simulink model "attsync2"  (R2013a)
settings: Solver=ode45  StartTime=0.0  StopTime=30  RelTol=1e-3
settings Model: Creator=daqing_yi  LastModifiedBy=daqing_yi
settings DataIOCC: SignalLoggingSaveFormat=ModelDataLogs
settings DebuggingCC: MultiTaskDSMMsg=warning  MultiTaskCondExecSysMsg=none  StrictBusMsg=None
settings RTWCC: IncludeERTFirstTime=on

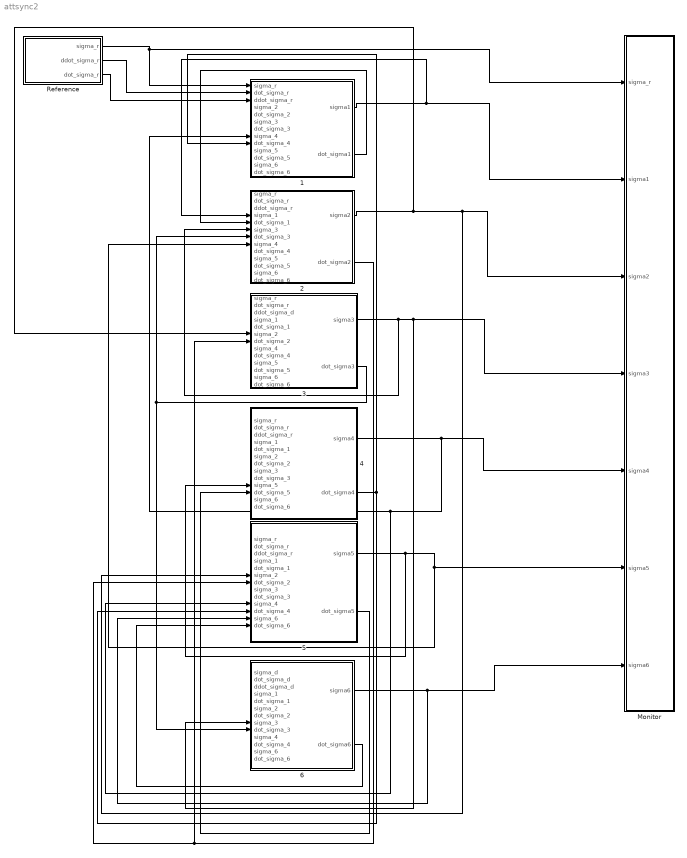
== system attsync2 ==
  1 : Subsystem
  2 : Subsystem
  3 : Subsystem
  4 : Subsystem
  5 : Subsystem
  6 : Subsystem
  Monitor : Subsystem
  Reference : Subsystem
  wires:
  Reference/1(sigma_r) -> 1/1(sigma_r), Monitor/1(sigma_r)
  1/1(sigma1) -> 2/4(sigma_1), Monitor/2(sigma1)
  2/1(sigma2) -> 3/6(sigma_2), 5/6(sigma_2), Monitor/3(sigma2)
  3/1(sigma3) -> 6/8(sigma_3), Monitor/4(sigma3), 2/6(sigma_3)
  4/1(sigma4) -> Monitor/5(sigma4), 5/10(sigma_4), 1/8(sigma_4)
  5/1(sigma5) -> 2/8(sigma_4), Monitor/6(sigma5), 4/10(sigma_5)
  Reference/2(ddot_sigma_r) -> 1/2(dot_sigma_r)
  Reference/3(dot_sigma_r) -> 1/3(ddot_sigma_r)
  6/1(sigma6) -> Monitor/7(sigma6), 5/12(sigma_6)
  6/2(dot_sigma6) -> 5/13(dot_sigma_6)
  3/2(dot_sigma3) -> 6/9(dot_sigma_3), 2/7(dot_sigma_3)
  4/2(dot_sigma4) -> 1/9(dot_sigma_4), 5/11(dot_sigma_4)
  5/2(dot_sigma5) -> 4/11(dot_sigma_5)
  2/2(dot_sigma2) -> 3/7(dot_sigma_2), 5/7(dot_sigma_2)
  1/2(dot_sigma1) -> 2/5(dot_sigma_1)

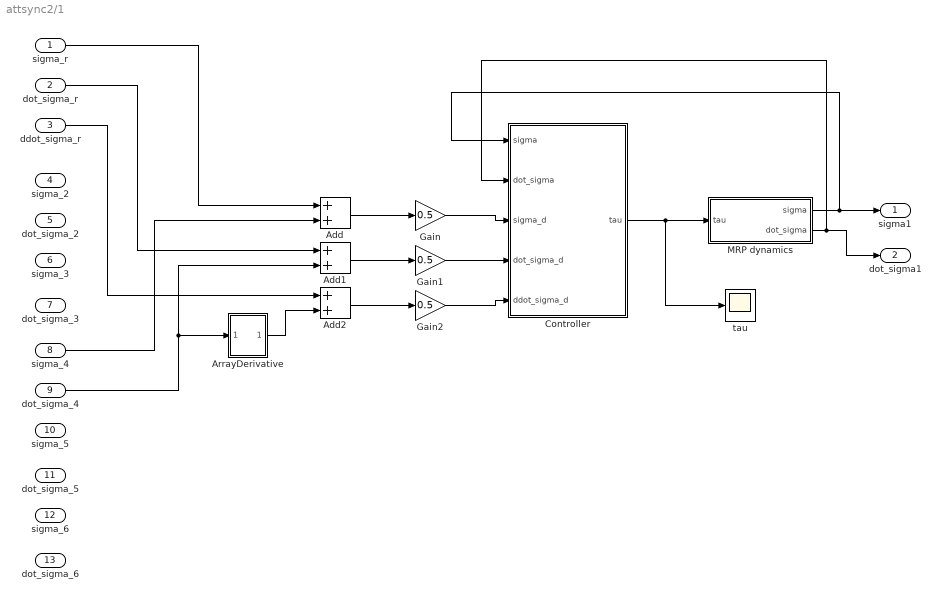
== system attsync2/1 ==
  sigma_r : Inport
  dot_sigma_r : Inport  Port=2
  ddot_sigma_r : Inport  Port=3
  sigma_2 : Inport  Port=4  PortDimensions=3
  dot_sigma_2 : Inport  Port=5  PortDimensions=3
  sigma_3 : Inport  Port=6  PortDimensions=3
  dot_sigma_3 : Inport  Port=7  PortDimensions=3
  sigma_4 : Inport  Port=8  PortDimensions=3
  dot_sigma_4 : Inport  Port=9  PortDimensions=3
  sigma_5 : Inport  Port=10  PortDimensions=3
  dot_sigma_5 : Inport  Port=11  PortDimensions=3
  sigma_6 : Inport  Port=12  PortDimensions=3
  dot_sigma_6 : Inport  Port=13  PortDimensions=3
  Add : Sum
  Add1 : Sum
  Add2 : Sum
  ArrayDerivative : Subsystem
  Controller : Subsystem
  Gain : Gain  Gain=0.5
  Gain1 : Gain  Gain=0.5
  Gain2 : Gain  Gain=0.5
  MRP dynamics : Subsystem
  tau : Scope
  sigma1 : Outport
  dot_sigma1 : Outport  Port=2
  wires:
  Controller/1(tau) -> tau/1, MRP dynamics/1(tau)
  MRP dynamics/1(sigma) -> sigma1/1, Controller/1(sigma)
  MRP dynamics/2(dot_sigma) -> dot_sigma1/1, Controller/2(dot_sigma)
  Add/1 -> Gain/1
  Add1/1 -> Gain1/1
  Add2/1 -> Gain2/1
  Gain/1 -> Controller/3(sigma_d)
  Gain1/1 -> Controller/4(dot_sigma_d)
  Gain2/1 -> Controller/5(ddot_sigma_d)
  sigma_r/1 -> Add/1
  dot_sigma_r/1 -> Add1/1
  ddot_sigma_r/1 -> Add2/1
  sigma_4/1 -> Add/2
  dot_sigma_4/1 -> Add1/2, ArrayDerivative/1(In1)
  ArrayDerivative/1(Out1) -> Add2/2

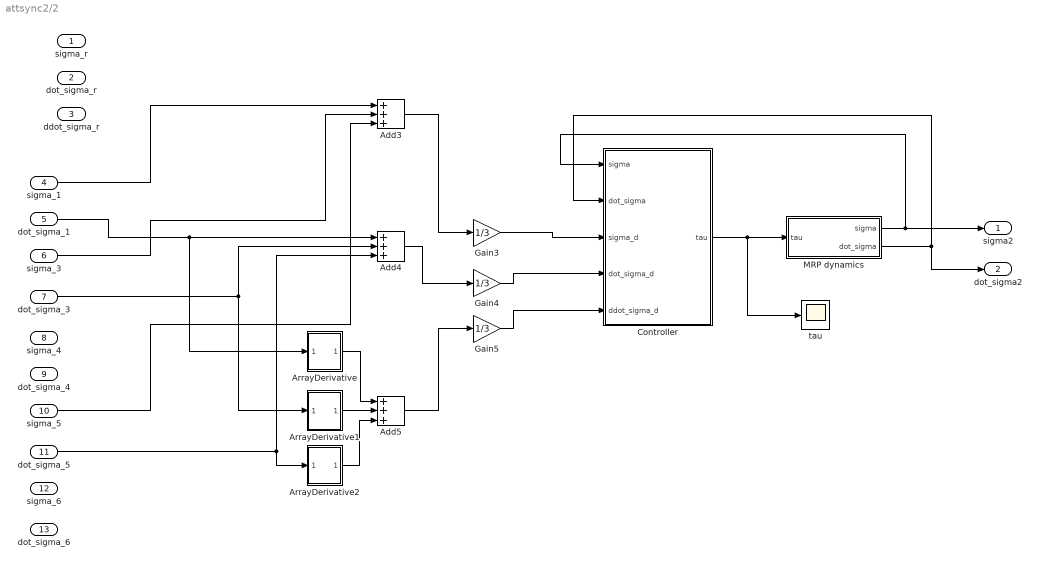
== system attsync2/2 ==
  sigma_r : Inport
  dot_sigma_r : Inport  Port=2
  ddot_sigma_r : Inport  Port=3
  sigma_1 : Inport  Port=4  PortDimensions=3
  dot_sigma_1 : Inport  Port=5  PortDimensions=3
  sigma_3 : Inport  Port=6  PortDimensions=3
  dot_sigma_3 : Inport  Port=7  PortDimensions=3
  sigma_4 : Inport  Port=8  PortDimensions=3
  dot_sigma_4 : Inport  Port=9  PortDimensions=3
  sigma_5 : Inport  Port=10  PortDimensions=3
  dot_sigma_5 : Inport  Port=11  PortDimensions=3
  sigma_6 : Inport  Port=12  PortDimensions=3
  dot_sigma_6 : Inport  Port=13  PortDimensions=3
  Add3 : Sum  Inputs=+++
  Add4 : Sum  Inputs=+++
  Add5 : Sum  Inputs=+++
  ArrayDerivative : Subsystem
  ArrayDerivative1 : Subsystem
  ArrayDerivative2 : Subsystem
  Controller : Subsystem
  Gain3 : Gain  Gain=1/3
  Gain4 : Gain  Gain=1/3
  Gain5 : Gain  Gain=1/3
  MRP dynamics : Subsystem
  tau : Scope
  sigma2 : Outport
  dot_sigma2 : Outport  Port=2
  wires:
  Controller/1(tau) -> tau/1, MRP dynamics/1(tau)
  MRP dynamics/1(sigma) -> sigma2/1, Controller/1(sigma)
  MRP dynamics/2(dot_sigma) -> dot_sigma2/1, Controller/2(dot_sigma)
  Add4/1 -> Gain4/1
  Add3/1 -> Gain3/1
  Gain3/1 -> Controller/3(sigma_d)
  Gain4/1 -> Controller/4(dot_sigma_d)
  Add5/1 -> Gain5/1
  Gain5/1 -> Controller/5(ddot_sigma_d)
  sigma_1/1 -> Add3/1
  sigma_3/1 -> Add3/2
  sigma_5/1 -> Add3/3
  dot_sigma_5/1 -> ArrayDerivative2/1(In1), Add4/3
  dot_sigma_1/1 -> ArrayDerivative/1(In1), Add4/1
  dot_sigma_3/1 -> ArrayDerivative1/1(In1), Add4/2
  ArrayDerivative2/1(Out1) -> Add5/3
  ArrayDerivative1/1(Out1) -> Add5/2
  ArrayDerivative/1(Out1) -> Add5/1

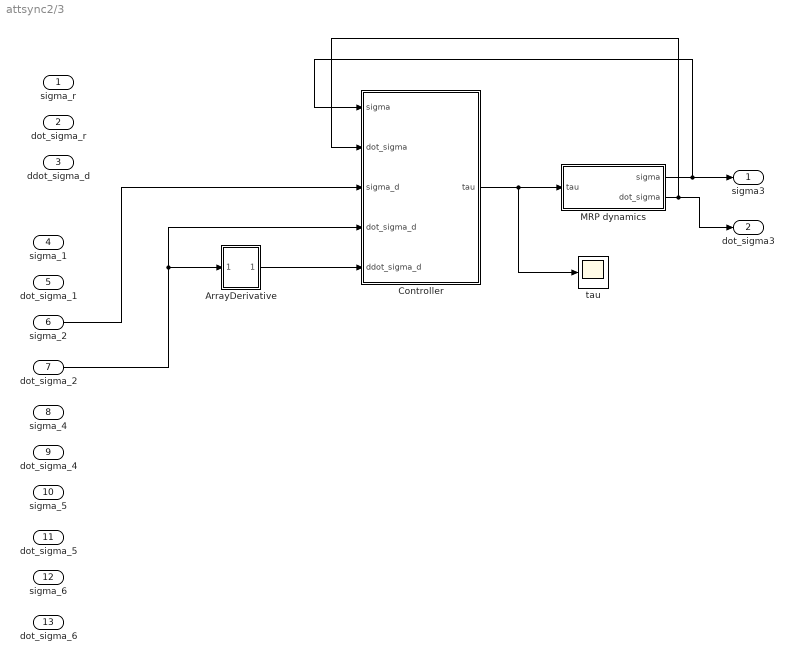
== system attsync2/3 ==
  sigma_r : Inport
  dot_sigma_r : Inport  Port=2
  ddot_sigma_d : Inport  Port=3
  sigma_1 : Inport  Port=4  PortDimensions=3
  dot_sigma_1 : Inport  Port=5  PortDimensions=3
  sigma_2 : Inport  Port=6  PortDimensions=3
  dot_sigma_2 : Inport  Port=7  PortDimensions=3
  sigma_4 : Inport  Port=8  PortDimensions=3
  dot_sigma_4 : Inport  Port=9  PortDimensions=3
  sigma_5 : Inport  Port=10  PortDimensions=3
  dot_sigma_5 : Inport  Port=11  PortDimensions=3
  sigma_6 : Inport  Port=12  PortDimensions=3
  dot_sigma_6 : Inport  Port=13  PortDimensions=3
  ArrayDerivative : Subsystem
  Controller : Subsystem
  MRP dynamics : Subsystem
  tau : Scope
  sigma3 : Outport
  dot_sigma3 : Outport  Port=2
  wires:
  Controller/1(tau) -> tau/1, MRP dynamics/1(tau)
  MRP dynamics/1(sigma) -> sigma3/1, Controller/1(sigma)
  MRP dynamics/2(dot_sigma) -> dot_sigma3/1, Controller/2(dot_sigma)
  sigma_2/1 -> Controller/3(sigma_d)
  dot_sigma_2/1 -> ArrayDerivative/1(In1), Controller/4(dot_sigma_d)
  ArrayDerivative/1(Out1) -> Controller/5(ddot_sigma_d)

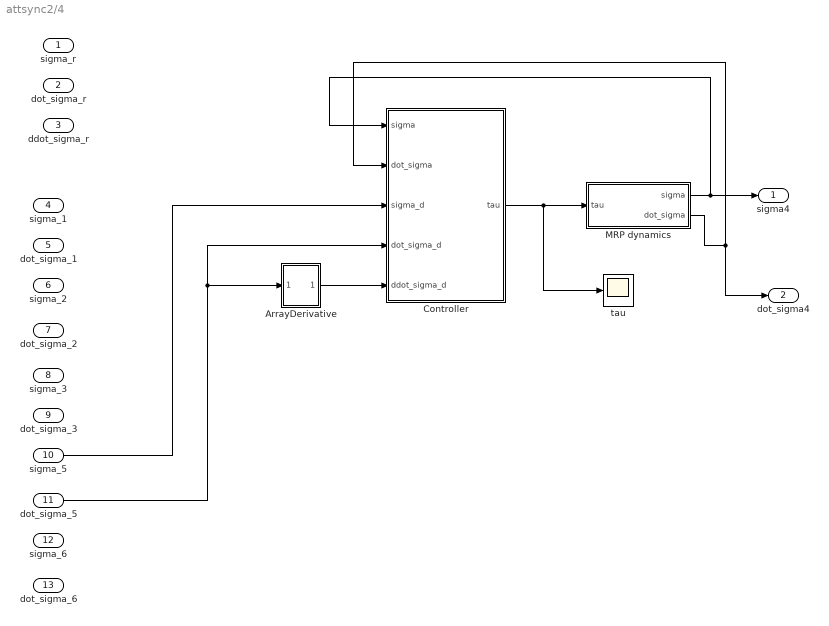
== system attsync2/4 ==
  sigma_r : Inport
  dot_sigma_r : Inport  Port=2
  ddot_sigma_r : Inport  Port=3
  sigma_1 : Inport  Port=4  PortDimensions=3
  dot_sigma_1 : Inport  Port=5  PortDimensions=3
  sigma_2 : Inport  Port=6  PortDimensions=3
  dot_sigma_2 : Inport  Port=7  PortDimensions=3
  sigma_3 : Inport  Port=8  PortDimensions=3
  dot_sigma_3 : Inport  Port=9  PortDimensions=3
  sigma_5 : Inport  Port=10  PortDimensions=3
  dot_sigma_5 : Inport  Port=11  PortDimensions=3
  sigma_6 : Inport  Port=12  PortDimensions=3
  dot_sigma_6 : Inport  Port=13  PortDimensions=3
  ArrayDerivative : Subsystem
  Controller : Subsystem
  MRP dynamics : Subsystem
  tau : Scope
  sigma4 : Outport
  dot_sigma4 : Outport  Port=2
  wires:
  Controller/1(tau) -> tau/1, MRP dynamics/1(tau)
  MRP dynamics/1(sigma) -> sigma4/1, Controller/1(sigma)
  MRP dynamics/2(dot_sigma) -> Controller/2(dot_sigma), dot_sigma4/1
  sigma_5/1 -> Controller/3(sigma_d)
  dot_sigma_5/1 -> ArrayDerivative/1(In1), Controller/4(dot_sigma_d)
  ArrayDerivative/1(Out1) -> Controller/5(ddot_sigma_d)

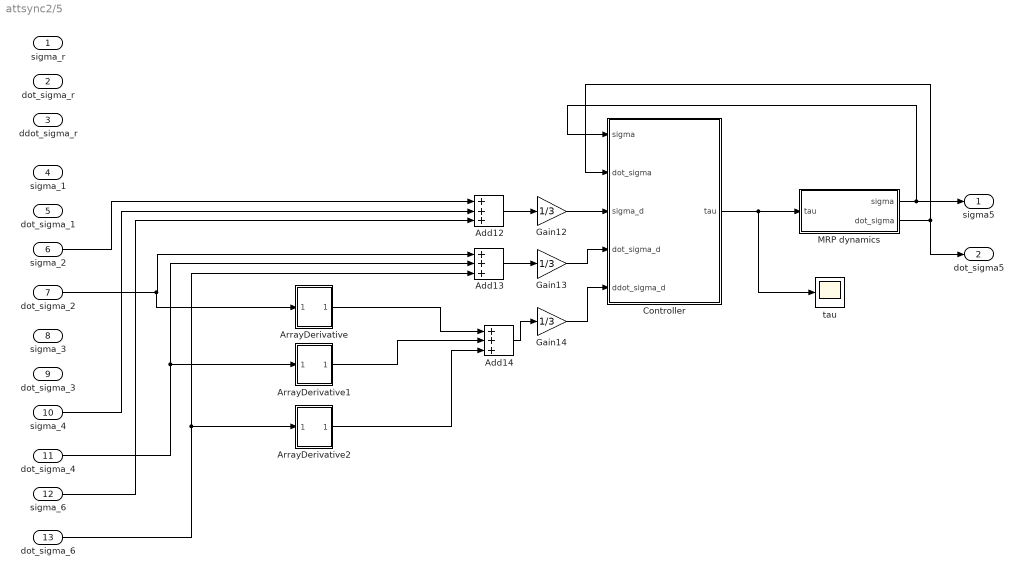
== system attsync2/5 ==
  sigma_r : Inport
  dot_sigma_r : Inport  Port=2
  ddot_sigma_r : Inport  Port=3
  sigma_1 : Inport  Port=4  PortDimensions=3
  dot_sigma_1 : Inport  Port=5  PortDimensions=3
  sigma_2 : Inport  Port=6  PortDimensions=3
  dot_sigma_2 : Inport  Port=7  PortDimensions=3
  sigma_3 : Inport  Port=8  PortDimensions=3
  dot_sigma_3 : Inport  Port=9  PortDimensions=3
  sigma_4 : Inport  Port=10  PortDimensions=3
  dot_sigma_4 : Inport  Port=11  PortDimensions=3
  sigma_6 : Inport  Port=12  PortDimensions=3
  dot_sigma_6 : Inport  Port=13  PortDimensions=3
  Add12 : Sum  Inputs=+++
  Add13 : Sum  Inputs=+++
  Add14 : Sum  Inputs=+++
  ArrayDerivative : Subsystem
  ArrayDerivative1 : Subsystem
  ArrayDerivative2 : Subsystem
  Controller : Subsystem
  Gain12 : Gain  Gain=1/3
  Gain13 : Gain  Gain=1/3
  Gain14 : Gain  Gain=1/3
  MRP dynamics : Subsystem
  tau : Scope
  sigma5 : Outport
  dot_sigma5 : Outport  Port=2
  wires:
  Controller/1(tau) -> tau/1, MRP dynamics/1(tau)
  MRP dynamics/1(sigma) -> sigma5/1, Controller/1(sigma)
  MRP dynamics/2(dot_sigma) -> dot_sigma5/1, Controller/2(dot_sigma)
  Add12/1 -> Gain12/1
  Add13/1 -> Gain13/1
  Add14/1 -> Gain14/1
  Gain12/1 -> Controller/3(sigma_d)
  Gain13/1 -> Controller/4(dot_sigma_d)
  Gain14/1 -> Controller/5(ddot_sigma_d)
  sigma_2/1 -> Add12/1
  sigma_4/1 -> Add12/2
  sigma_6/1 -> Add12/3
  dot_sigma_2/1 -> ArrayDerivative/1(In1), Add13/1
  dot_sigma_4/1 -> ArrayDerivative1/1(In1), Add13/2
  dot_sigma_6/1 -> ArrayDerivative2/1(In1), Add13/3
  ArrayDerivative1/1(Out1) -> Add14/2
  ArrayDerivative2/1(Out1) -> Add14/3
  ArrayDerivative/1(Out1) -> Add14/1

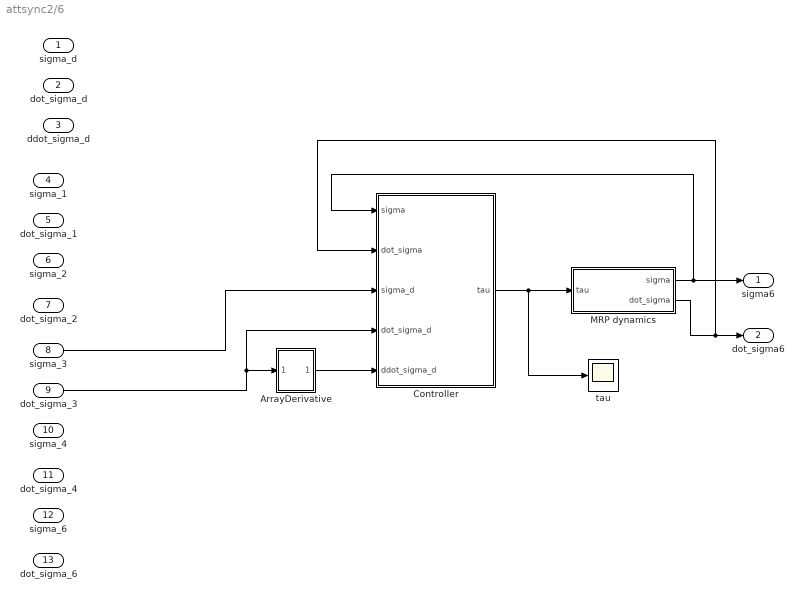
== system attsync2/6 ==
  sigma_d : Inport
  dot_sigma_d : Inport  Port=2
  ddot_sigma_d : Inport  Port=3
  sigma_1 : Inport  Port=4  PortDimensions=3
  dot_sigma_1 : Inport  Port=5  PortDimensions=3
  sigma_2 : Inport  Port=6  PortDimensions=3
  dot_sigma_2 : Inport  Port=7  PortDimensions=3
  sigma_3 : Inport  Port=8  PortDimensions=3
  dot_sigma_3 : Inport  Port=9  PortDimensions=3
  sigma_4 : Inport  Port=10  PortDimensions=3
  dot_sigma_4 : Inport  Port=11  PortDimensions=3
  sigma_6 : Inport  Port=12  PortDimensions=3
  dot_sigma_6 : Inport  Port=13  PortDimensions=3
  ArrayDerivative : Subsystem
  Controller : Subsystem
  MRP dynamics : Subsystem
  tau : Scope
  sigma6 : Outport
  dot_sigma6 : Outport  Port=2
  wires:
  Controller/1(tau) -> tau/1, MRP dynamics/1(tau)
  MRP dynamics/1(sigma) -> sigma6/1, Controller/1(sigma)
  MRP dynamics/2(dot_sigma) -> Controller/2(dot_sigma), dot_sigma6/1
  sigma_3/1 -> Controller/3(sigma_d)
  dot_sigma_3/1 -> ArrayDerivative/1(In1), Controller/4(dot_sigma_d)
  ArrayDerivative/1(Out1) -> Controller/5(ddot_sigma_d)

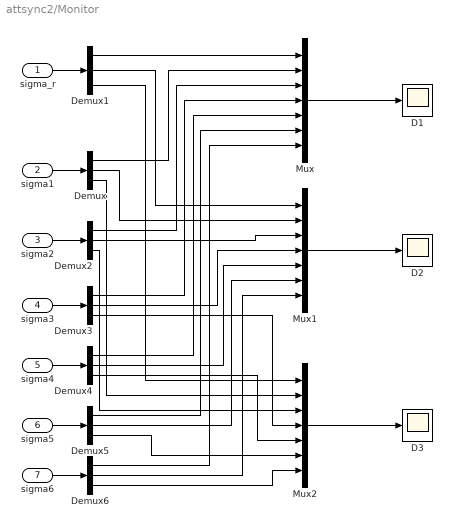
== system attsync2/Monitor ==
  sigma_r : Inport
  sigma1 : Inport  Port=2
  sigma2 : Inport  Port=3
  sigma3 : Inport  Port=4
  sigma4 : Inport  Port=5
  sigma5 : Inport  Port=6
  sigma6 : Inport  Port=7
  D1 : Scope
      settings: YMin=-8  YMax=1.5  SaveName=D1
  D2 : Scope
      settings: SaveName=D2
  D3 : Scope
      settings: SaveName=D3
  Demux{,1..6} (7 alike) : Demux  Outputs=3
  Mux : Mux  Inputs=7
  Mux1 : Mux  Inputs=7
  Mux2 : Mux  Inputs=7
  wires:
  sigma1/1 -> Demux/1
  sigma_r/1 -> Demux1/1
  Demux1/1 -> Mux/1
  Mux/1 -> D1/1
  Mux1/1 -> D2/1
  Mux2/1 -> D3/1
  sigma3/1 -> Demux3/1
  sigma4/1 -> Demux4/1
  sigma5/1 -> Demux5/1
  sigma6/1 -> Demux6/1
  sigma2/1 -> Demux2/1
  Demux1/2 -> Mux1/1
  Demux1/3 -> Mux2/1
  Demux/1 -> Mux/2
  Demux2/1 -> Mux/3
  Demux3/1 -> Mux/4
  Demux4/1 -> Mux/5
  Demux5/1 -> Mux/6
  Demux6/1 -> Mux/7
  Demux/2 -> Mux1/2
  Demux2/2 -> Mux1/3
  Demux3/2 -> Mux1/4
  Demux4/2 -> Mux1/5
  Demux5/2 -> Mux1/6
  Demux6/2 -> Mux1/7
  Demux/3 -> Mux2/2
  Demux2/3 -> Mux2/3
  Demux3/3 -> Mux2/4
  Demux4/3 -> Mux2/5
  Demux5/3 -> Mux2/6
  Demux6/3 -> Mux2/7

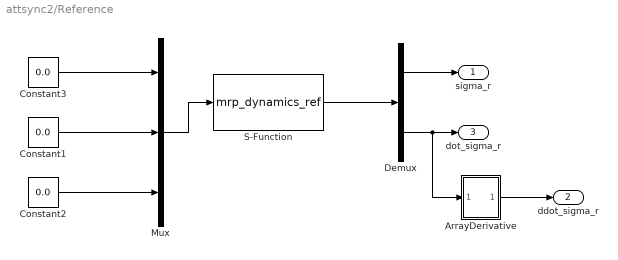
== system attsync2/Reference ==
  ArrayDerivative : Subsystem
  Constant1 : Constant  Value=0.0
  Constant2 : Constant  Value=0.0
  Constant3 : Constant  Value=0.0
  Demux : Demux  Outputs=2
  Mux : Mux  Inputs=3
  S-Function : S-Function  FunctionName=mrp_dynamics_ref  EnableBusSupport=off
  sigma_r : Outport  PortDimensions=3
  ddot_sigma_r : Outport  Port=2
  dot_sigma_r : Outport  Port=3
  wires:
  Constant3/1 -> Mux/1
  Constant1/1 -> Mux/2
  Constant2/1 -> Mux/3
  Mux/1 -> S-Function/1
  S-Function/1 -> Demux/1
  Demux/1 -> sigma_r/1
  Demux/2 -> ArrayDerivative/1(In1), dot_sigma_r/1
  ArrayDerivative/1(Out1) -> ddot_sigma_r/1

== system attsync2/1/ArrayDerivative ==
  In1 : Inport
  Demux : Demux  Outputs=3
  Derivative : Derivative
  Derivative1 : Derivative
  Derivative2 : Derivative
  Mux : Mux  Inputs=3
  Out1 : Outport
  wires:
  Mux/1 -> Out1/1
  In1/1 -> Demux/1
  Derivative1/1 -> Mux/2
  Demux/2 -> Derivative1/1
  Derivative2/1 -> Mux/3
  Demux/3 -> Derivative2/1
  Demux/1 -> Derivative/1
  Derivative/1 -> Mux/1

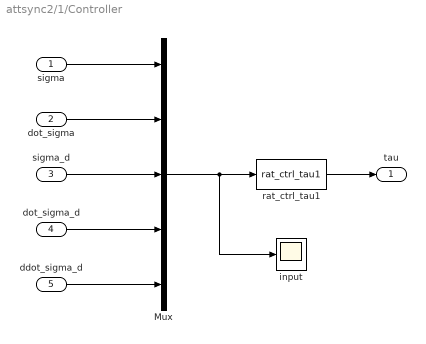
== system attsync2/1/Controller ==
  sigma : Inport
  dot_sigma : Inport  Port=2
  sigma_d : Inport  Port=3
  dot_sigma_d : Inport  Port=4
  ddot_sigma_d : Inport  Port=5
  Mux : Mux  Inputs=5
  input : Scope
      settings: SaveName=ScopeData4
  rat_ctrl_tau1 : MATLABFcn  MATLABFcn=rat_ctrl_tau1  OutputDimensions=3
  tau : Outport
  wires:
  sigma/1 -> Mux/1
  sigma_d/1 -> Mux/3
  Mux/1 -> input/1, rat_ctrl_tau1/1
  dot_sigma/1 -> Mux/2
  rat_ctrl_tau1/1 -> tau/1
  dot_sigma_d/1 -> Mux/4
  ddot_sigma_d/1 -> Mux/5

== system attsync2/1/MRP dynamics ==
  tau : Inport
  Demux : Demux  Outputs=2
  S-Function : S-Function  FunctionName=mrp_dynamics1  EnableBusSupport=off
  sigma : Outport  PortDimensions=3
  dot_sigma : Outport  Port=2  PortDimensions=3
  wires:
  tau/1 -> S-Function/1
  Demux/1 -> sigma/1
  Demux/2 -> dot_sigma/1
  S-Function/1 -> Demux/1

== system attsync2/2/ArrayDerivative ==
  In1 : Inport
  Demux : Demux  Outputs=3
  Derivative : Derivative
  Derivative1 : Derivative
  Derivative2 : Derivative
  Mux : Mux  Inputs=3
  Out1 : Outport
  wires:
  Mux/1 -> Out1/1
  In1/1 -> Demux/1
  Derivative1/1 -> Mux/2
  Demux/2 -> Derivative1/1
  Derivative2/1 -> Mux/3
  Demux/3 -> Derivative2/1
  Demux/1 -> Derivative/1
  Derivative/1 -> Mux/1

== system attsync2/2/ArrayDerivative1 ==
  In1 : Inport
  Demux : Demux  Outputs=3
  Derivative : Derivative
  Derivative1 : Derivative
  Derivative2 : Derivative
  Mux : Mux  Inputs=3
  Out1 : Outport
  wires:
  Mux/1 -> Out1/1
  In1/1 -> Demux/1
  Derivative1/1 -> Mux/2
  Demux/2 -> Derivative1/1
  Derivative2/1 -> Mux/3
  Demux/3 -> Derivative2/1
  Demux/1 -> Derivative/1
  Derivative/1 -> Mux/1

== system attsync2/2/ArrayDerivative2 ==
  In1 : Inport
  Demux : Demux  Outputs=3
  Derivative : Derivative
  Derivative1 : Derivative
  Derivative2 : Derivative
  Mux : Mux  Inputs=3
  Out1 : Outport
  wires:
  Mux/1 -> Out1/1
  In1/1 -> Demux/1
  Derivative1/1 -> Mux/2
  Demux/2 -> Derivative1/1
  Derivative2/1 -> Mux/3
  Demux/3 -> Derivative2/1
  Demux/1 -> Derivative/1
  Derivative/1 -> Mux/1

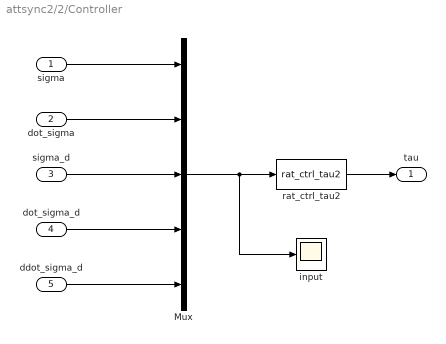
== system attsync2/2/Controller ==
  sigma : Inport
  dot_sigma : Inport  Port=2
  sigma_d : Inport  Port=3
  dot_sigma_d : Inport  Port=4
  ddot_sigma_d : Inport  Port=5
  Mux : Mux  Inputs=5
  input : Scope
      settings: SaveName=ScopeData4
  rat_ctrl_tau2 : MATLABFcn  MATLABFcn=rat_ctrl_tau2  OutputDimensions=3
  tau : Outport
  wires:
  sigma/1 -> Mux/1
  sigma_d/1 -> Mux/3
  Mux/1 -> input/1, rat_ctrl_tau2/1
  dot_sigma/1 -> Mux/2
  rat_ctrl_tau2/1 -> tau/1
  dot_sigma_d/1 -> Mux/4
  ddot_sigma_d/1 -> Mux/5

== system attsync2/2/MRP dynamics ==
  tau : Inport
  Demux : Demux  Outputs=2
  S-Function : S-Function  FunctionName=mrp_dynamics2  EnableBusSupport=off
  sigma : Outport  PortDimensions=3
  dot_sigma : Outport  Port=2  PortDimensions=3
  wires:
  tau/1 -> S-Function/1
  Demux/1 -> sigma/1
  Demux/2 -> dot_sigma/1
  S-Function/1 -> Demux/1

== system attsync2/3/ArrayDerivative ==
  In1 : Inport
  Demux : Demux  Outputs=3
  Derivative : Derivative
  Derivative1 : Derivative
  Derivative2 : Derivative
  Mux : Mux  Inputs=3
  Out1 : Outport
  wires:
  Mux/1 -> Out1/1
  In1/1 -> Demux/1
  Derivative1/1 -> Mux/2
  Demux/2 -> Derivative1/1
  Derivative2/1 -> Mux/3
  Demux/3 -> Derivative2/1
  Demux/1 -> Derivative/1
  Derivative/1 -> Mux/1

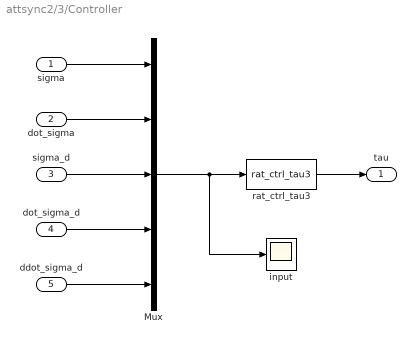
== system attsync2/3/Controller ==
  sigma : Inport  PortDimensions=3
  dot_sigma : Inport  Port=2  PortDimensions=3
  sigma_d : Inport  Port=3  PortDimensions=3
  dot_sigma_d : Inport  Port=4  PortDimensions=3
  ddot_sigma_d : Inport  Port=5  PortDimensions=3
  Mux : Mux  Inputs=5
  input : Scope
      settings: SaveName=ScopeData4
  rat_ctrl_tau3 : MATLABFcn  MATLABFcn=rat_ctrl_tau3  OutputDimensions=3
  tau : Outport
  wires:
  sigma/1 -> Mux/1
  sigma_d/1 -> Mux/3
  Mux/1 -> input/1, rat_ctrl_tau3/1
  dot_sigma/1 -> Mux/2
  rat_ctrl_tau3/1 -> tau/1
  ddot_sigma_d/1 -> Mux/5
  dot_sigma_d/1 -> Mux/4

== system attsync2/3/MRP dynamics ==
  tau : Inport
  Demux : Demux  Outputs=2
  S-Function : S-Function  FunctionName=mrp_dynamics3  EnableBusSupport=off
  sigma : Outport  PortDimensions=3
  dot_sigma : Outport  Port=2  PortDimensions=3
  wires:
  S-Function/1 -> Demux/1
  tau/1 -> S-Function/1
  Demux/1 -> sigma/1
  Demux/2 -> dot_sigma/1

== system attsync2/4/ArrayDerivative ==
  In1 : Inport
  Demux : Demux  Outputs=3
  Derivative : Derivative
  Derivative1 : Derivative
  Derivative2 : Derivative
  Mux : Mux  Inputs=3
  Out1 : Outport
  wires:
  Mux/1 -> Out1/1
  In1/1 -> Demux/1
  Derivative1/1 -> Mux/2
  Demux/2 -> Derivative1/1
  Derivative2/1 -> Mux/3
  Demux/3 -> Derivative2/1
  Demux/1 -> Derivative/1
  Derivative/1 -> Mux/1

== system attsync2/4/Controller ==
  sigma : Inport
  dot_sigma : Inport  Port=2
  sigma_d : Inport  Port=3
  dot_sigma_d : Inport  Port=4
  ddot_sigma_d : Inport  Port=5
  Mux : Mux  Inputs=5
  input : Scope
      settings: SaveName=ScopeData4
  rat_ctrl_tau4 : MATLABFcn  MATLABFcn=rat_ctrl_tau4  OutputDimensions=3
  tau : Outport
  wires:
  sigma/1 -> Mux/1
  sigma_d/1 -> Mux/3
  Mux/1 -> input/1, rat_ctrl_tau4/1
  dot_sigma/1 -> Mux/2
  rat_ctrl_tau4/1 -> tau/1
  dot_sigma_d/1 -> Mux/4
  ddot_sigma_d/1 -> Mux/5

== system attsync2/4/MRP dynamics ==
  tau : Inport
  Demux : Demux  Outputs=2
  S-Function : S-Function  FunctionName=mrp_dynamics4  EnableBusSupport=off
  sigma : Outport  PortDimensions=3
  dot_sigma : Outport  Port=2  PortDimensions=3
  wires:
  S-Function/1 -> Demux/1
  tau/1 -> S-Function/1
  Demux/1 -> sigma/1
  Demux/2 -> dot_sigma/1

== system attsync2/5/ArrayDerivative ==
  In1 : Inport
  Demux : Demux  Outputs=3
  Derivative : Derivative
  Derivative1 : Derivative
  Derivative2 : Derivative
  Mux : Mux  Inputs=3
  Out1 : Outport
  wires:
  Mux/1 -> Out1/1
  In1/1 -> Demux/1
  Derivative1/1 -> Mux/2
  Demux/2 -> Derivative1/1
  Derivative2/1 -> Mux/3
  Demux/3 -> Derivative2/1
  Demux/1 -> Derivative/1
  Derivative/1 -> Mux/1

== system attsync2/5/ArrayDerivative1 ==
  In1 : Inport
  Demux : Demux  Outputs=3
  Derivative : Derivative
  Derivative1 : Derivative
  Derivative2 : Derivative
  Mux : Mux  Inputs=3
  Out1 : Outport
  wires:
  Mux/1 -> Out1/1
  In1/1 -> Demux/1
  Derivative1/1 -> Mux/2
  Demux/2 -> Derivative1/1
  Derivative2/1 -> Mux/3
  Demux/3 -> Derivative2/1
  Demux/1 -> Derivative/1
  Derivative/1 -> Mux/1

== system attsync2/5/ArrayDerivative2 ==
  In1 : Inport
  Demux : Demux  Outputs=3
  Derivative : Derivative
  Derivative1 : Derivative
  Derivative2 : Derivative
  Mux : Mux  Inputs=3
  Out1 : Outport
  wires:
  Mux/1 -> Out1/1
  In1/1 -> Demux/1
  Derivative1/1 -> Mux/2
  Demux/2 -> Derivative1/1
  Derivative2/1 -> Mux/3
  Demux/3 -> Derivative2/1
  Demux/1 -> Derivative/1
  Derivative/1 -> Mux/1

== system attsync2/5/Controller ==
  sigma : Inport
  dot_sigma : Inport  Port=2
  sigma_d : Inport  Port=3
  dot_sigma_d : Inport  Port=4
  ddot_sigma_d : Inport  Port=5
  Mux : Mux  Inputs=5
  input : Scope
      settings: SaveName=ScopeData4
  rat_ctrl_tau5 : MATLABFcn  MATLABFcn=rat_ctrl_tau5  OutputDimensions=3
  tau : Outport
  wires:
  sigma/1 -> Mux/1
  sigma_d/1 -> Mux/3
  Mux/1 -> input/1, rat_ctrl_tau5/1
  dot_sigma/1 -> Mux/2
  rat_ctrl_tau5/1 -> tau/1
  dot_sigma_d/1 -> Mux/4
  ddot_sigma_d/1 -> Mux/5

== system attsync2/5/MRP dynamics ==
  tau : Inport
  Demux : Demux  Outputs=2
  S-Function : S-Function  FunctionName=mrp_dynamics5  EnableBusSupport=off
  sigma : Outport  PortDimensions=3
  dot_sigma : Outport  Port=2  PortDimensions=3
  wires:
  S-Function/1 -> Demux/1
  tau/1 -> S-Function/1
  Demux/1 -> sigma/1
  Demux/2 -> dot_sigma/1

== system attsync2/6/ArrayDerivative ==
  In1 : Inport
  Demux : Demux  Outputs=3
  Derivative : Derivative
  Derivative1 : Derivative
  Derivative2 : Derivative
  Mux : Mux  Inputs=3
  Out1 : Outport
  wires:
  Mux/1 -> Out1/1
  In1/1 -> Demux/1
  Derivative1/1 -> Mux/2
  Demux/2 -> Derivative1/1
  Derivative2/1 -> Mux/3
  Demux/3 -> Derivative2/1
  Demux/1 -> Derivative/1
  Derivative/1 -> Mux/1

== system attsync2/6/Controller ==
  sigma : Inport
  dot_sigma : Inport  Port=2
  sigma_d : Inport  Port=3
  dot_sigma_d : Inport  Port=4
  ddot_sigma_d : Inport  Port=5
  Mux : Mux  Inputs=5
  input : Scope
      settings: SaveName=ScopeData4
  rat_ctrl_tau6 : MATLABFcn  MATLABFcn=rat_ctrl_tau6  OutputDimensions=3
  tau : Outport
  wires:
  sigma/1 -> Mux/1
  sigma_d/1 -> Mux/3
  Mux/1 -> input/1, rat_ctrl_tau6/1
  dot_sigma/1 -> Mux/2
  rat_ctrl_tau6/1 -> tau/1
  dot_sigma_d/1 -> Mux/4
  ddot_sigma_d/1 -> Mux/5

== system attsync2/6/MRP dynamics ==
  tau : Inport
  Demux : Demux  Outputs=2
  S-Function : S-Function  FunctionName=mrp_dynamics6  EnableBusSupport=off
  sigma : Outport  PortDimensions=3
  dot_sigma : Outport  Port=2  PortDimensions=3
  wires:
  S-Function/1 -> Demux/1
  tau/1 -> S-Function/1
  Demux/1 -> sigma/1
  Demux/2 -> dot_sigma/1

== system attsync2/Reference/ArrayDerivative ==
  In1 : Inport
  Demux : Demux  Outputs=3
  Derivative : Derivative
  Derivative1 : Derivative
  Derivative2 : Derivative
  Mux : Mux  Inputs=3
  Out1 : Outport
  wires:
  Mux/1 -> Out1/1
  In1/1 -> Demux/1
  Derivative1/1 -> Mux/2
  Demux/2 -> Derivative1/1
  Derivative2/1 -> Mux/3
  Demux/3 -> Derivative2/1
  Demux/1 -> Derivative/1
  Derivative/1 -> Mux/1
